simulink model "Scissor_Lift_4_Hydraulic_Actuator"  (Simulink 7.9)
settings: Solver=ode15s  StartTime=0.0  StopTime=10.0  MaxStep=1e-2  RelTol=1e-3  AbsTol=1e-4
PostLoadFcn:
  | warning off Simulink:Engine:OutputNotConnected
  | warning off mech2:compiler:topologyAnalysis:DanglingBlock
undefined symbols (not defined in the file): Local, Scissor_Lift_Param, X, Y, Z
libraries: sm_lib x48, Scissor_Parts_Lib x21, fl_lib x8, nesl_utility x7, sh_lib x4
(part 2 of 2)

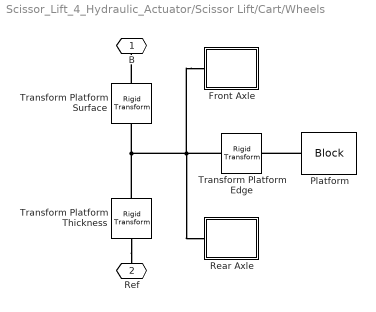
== system Scissor_Lift_4_Hydraulic_Actuator/Scissor Lift/Cart/Wheels ==
  Front Axle : Subsystem
  Platform : Scissor_Parts_Lib/Block  L=Scissor_Lift_Param.Cart.Platform.Width  W=Scissor_Lift_Param.Cart.Platform.Length  H=Scissor_Lift_Param.Cart.Platform.Height  z_ori=Local +Z  rho=Scissor_Lift_Param.Base_Block.Density  clr=Scissor_Lift_Param.Base_Block.Color  opc=Scissor_Lift_Param.Base_Block.Opacity
  Rear Axle : Subsystem
  Transform Platform Surface : sm_lib/Frames and  Transforms/Rigid  Transform  TranslationMethod=Cartesian  TranslationLengthUnit=cm  TranslationStandardAxis=+Y  TranslationStandardOffset=Scissor_Lift_Param.Cart.Platform.Height/2  TranslationCartesianOffset=[0 Scissor_Lift_Param.Cart.Platform.Height/2 0]  TranslationROffset=0  TranslationROffsetUnits=m  TranslationZOffset=0  TranslationZOffsetUnits=m  TranslationThetaOffset=0  TranslationThetaOffsetUnits=deg  RotationMethod=None  RotationAngleUnits=deg  RotationStandardAxis=+X  RotationAngle=90  RotationArbitraryAxis=[0 0 1]  FollAlignAxisA=+X  BaseAlignAxisA=+Y  FollAlignAxisB=+Y  BaseAlignAxisB=+Z  BlockFunction=simmechanics.library.frames_transforms.rigid_transform
  Transform Platform Thickness : sm_lib/Frames and  Transforms/Rigid  Transform  TranslationMethod=StandardAxis  TranslationLengthUnit=cm  TranslationStandardAxis=+Z  TranslationStandardOffset=Scissor_Lift_Param.Cart.Platform.Height/2  TranslationCartesianOffset=[0 0 0]  TranslationROffset=0  TranslationROffsetUnits=m  TranslationZOffset=0  TranslationZOffsetUnits=m  TranslationThetaOffset=0  TranslationThetaOffsetUnits=deg  RotationMethod=StandardAxis  RotationAngleUnits=deg  RotationStandardAxis=+X  RotationAngle=90  RotationArbitraryAxis=[0 0 1]  FollAlignAxisA=+X  BaseAlignAxisA=+Y  FollAlignAxisB=+Y  BaseAlignAxisB=+Z  BlockFunction=simmechanics.library.frames_transforms.rigid_transform
  Transform Platform Edge : sm_lib/Frames and  Transforms/Rigid  Transform  TranslationMethod=Cartesian  TranslationLengthUnit=cm  TranslationStandardAxis=+Z  TranslationStandardOffset=0  TranslationCartesianOffset=[Scissor_Lift_Param.Cart.Platform.Length 0 -Scissor_Lift_Param.Cart.Platform.Width]/2  TranslationROffset=0  TranslationROffsetUnits=m  TranslationZOffset=0  TranslationZOffsetUnits=m  TranslationThetaOffset=0  TranslationThetaOffsetUnits=deg  RotationMethod=None  RotationAngleUnits=deg  RotationStandardAxis=+X  RotationAngle=90  RotationArbitraryAxis=[0 0 1]  FollAlignAxisA=+X  BaseAlignAxisA=+Y  FollAlignAxisB=+Y  BaseAlignAxisB=+Z  BlockFunction=simmechanics.library.frames_transforms.rigid_transform
  " B" : PMIOPort  Port=1  Side=Right
  Ref : PMIOPort  Port=2  Side=Left
  connections:
  Transform Platform Surface/RConn1 -- " B"/RConn1
  Transform Platform Thickness/LConn1 -- Ref/RConn1
  Platform/LConn1 -- Transform Platform Edge/RConn1
  Front Axle/LConn1 -- Rear Axle/LConn1 -- Transform Platform Surface/LConn1 -- Transform Platform Thickness/RConn1 -- Transform Platform Edge/LConn1

== system Scissor_Lift_4_Hydraulic_Actuator/Scissor Lift/Actuator/Actuator/MS2G Intf ==
  Ideal Force Sensor : fl_lib/Mechanical/Mechanical Sensors/Ideal Force Sensor  v_Log=off  f_Log=off  LocalVarNames=|v|f  LocalVarDescs=|v|f  LocalVarLogging=[0 0]
  Ideal Translational Velocity Source : fl_lib/Mechanical/Mechanical Sources/Ideal Translational Velocity Source  v_Log=off  f_Log=off  LocalVarNames=|v|f  LocalVarDescs=|v|f  LocalVarLogging=[0 0]
  V : PMIOPort  Port=1  Side=Left
  F : PMIOPort  Port=2  Side=Right
  R : PMIOPort  Port=3  Side=Left
  C : PMIOPort  Port=4  Side=Right
  connections:
  V/RConn1 -- Ideal Translational Velocity Source/RConn1
  F/RConn1 -- Ideal Force Sensor/RConn2
  Ideal Force Sensor/LConn1 -- Ideal Translational Velocity Source/RConn2
  R/RConn1 -- Ideal Translational Velocity Source/LConn1
  Ideal Force Sensor/RConn1 -- C/RConn1

== system Scissor_Lift_4_Hydraulic_Actuator/Scissor Lift/Cart/Wheels/Front Axle ==
  Axle : Subsystem  mask(Axle){Ra=Scissor_Lift_Param.Cart.Axle.Radius, Wd=Scissor_Lift_Param.Cart.Axle.Wheel_Distance, Rr=Scissor_Lift_Param.Cart.Axle.Rim.Radius, Tr=Scissor_Lift_Param.Cart.Axle.Rim.Thickness, rho=Scissor_Lift_Param.Cart.Axle.Rim.Density, clr=Scissor_Lift_Param.Cart.Axle.Rim.Color}
      mask prompts: Ra "Axle radius (cm)"; Wd "Wheel distance (cm)"; Rr "Rim radius (cm)"; Tr "Rim thickness (cm)"; rho "Density (kg/m^3)"; clr "Color"
      mask TabNameString: Dimensions,Dimensions,Dimensions,Dimensions,Material Properties,Material Properties
      mask Display:
      | image(imread('sm_wlandgear_axle.png'));
      | port_label('LConn',1,'M');
      | port_label('RConn',1,'L');
      | port_label('RConn',2,'R');
  Axle-Tire A Revolute : sm_lib/Joints/Revolute Joint  SenseConstraintForceX=off  SenseConstraintForceY=off  SenseConstraintForceZ=off  SenseConstraintTorqueX=off  SenseConstraintTorqueY=off  SenseConstraintTorqueZ=off  ConstraintWrenchDir=FollowerOnBase  ConstraintWrenchFrame=BaseFrame  EquilibriumPosition=0  EquilibriumPositionUnits=rad  SpringStiffness=0  SpringStiffnessUnits=N*m/rad  DampingCoefficient=0  DampingCoefficientUnits=N*m/(rad/s)  ActuationMode=NoActuation  SensePosition=off  SenseVelocity=off  SenseAcceleration=off  SenseTorqueForce=off  PositionTargetValue=0  PositionTargetValueUnits=rad  PositionTargetSpecify=off  PositionTargetPriority=High  VelocityTargetValue=0  VelocityTargetValueUnits=rad/s  VelocityTargetSpecify=off  VelocityTargetPriority=High  BlockFunction=simmechanics.library.joints.revolute_joint
  Axle-Tire B Revolute : sm_lib/Joints/Revolute Joint  SenseConstraintForceX=off  SenseConstraintForceY=off  SenseConstraintForceZ=off  SenseConstraintTorqueX=off  SenseConstraintTorqueY=off  SenseConstraintTorqueZ=off  ConstraintWrenchDir=FollowerOnBase  ConstraintWrenchFrame=BaseFrame  EquilibriumPosition=0  EquilibriumPositionUnits=rad  SpringStiffness=0  SpringStiffnessUnits=N*m/rad  DampingCoefficient=0  DampingCoefficientUnits=N*m/(rad/s)  ActuationMode=NoActuation  SensePosition=off  SenseVelocity=off  SenseAcceleration=off  SenseTorqueForce=off  PositionTargetValue=0  PositionTargetValueUnits=rad  PositionTargetSpecify=off  PositionTargetPriority=High  VelocityTargetValue=0  VelocityTargetValueUnits=rad/s  VelocityTargetSpecify=off  VelocityTargetPriority=High  BlockFunction=simmechanics.library.joints.revolute_joint
  Tire A : Subsystem  mask(Tire){Rt=Scissor_Lift_Param.Cart.Axle.Tire.Radius, Rr=Scissor_Lift_Param.Cart.Axle.Rim.Radius, Tt=Scissor_Lift_Param.Cart.Axle.Tire.Thickness, rho=Scissor_Lift_Param.Cart.Axle.Tire.Density, clr=Scissor_Lift_Param.Cart.Axle.Tire.Color}
      mask prompts: Rt "Tire radius (cm)"; Rr "Rim radius (cm)"; Tt "Tire thickness (cm)"; rho "Density (kg/m^3)"; clr "Color"
      mask init:
      | theta = [(0:1:359) 0]'*pi/180;
      | unit_circle = [cos(theta), sin(theta)];
      | tire_sec = [Rt * unit_circle; Rr * flipud(unit_circle)];
      mask TabNameString: Dimensions,Dimensions,Dimensions,Material Properties,Material Properties
      mask Display:
      | image(imread('sm_wlandgear_tire.png'));
      | port_label('LConn',1,'C');
  Tire B : Subsystem  mask(Tire){Rt=Scissor_Lift_Param.Cart.Axle.Tire.Radius, Rr=Scissor_Lift_Param.Cart.Axle.Rim.Radius, Tt=Scissor_Lift_Param.Cart.Axle.Tire.Thickness, rho=Scissor_Lift_Param.Cart.Axle.Tire.Density, clr=Scissor_Lift_Param.Cart.Axle.Tire.Color}
      mask prompts: Rt "Tire radius (cm)"; Rr "Rim radius (cm)"; Tt "Tire thickness (cm)"; rho "Density (kg/m^3)"; clr "Color"
      mask init:
      | theta = [(0:1:359) 0]'*pi/180;
      | unit_circle = [cos(theta), sin(theta)];
      | tire_sec = [Rt * unit_circle; Rr * flipud(unit_circle)];
      mask TabNameString: Dimensions,Dimensions,Dimensions,Material Properties,Material Properties
      mask Display:
      | image(imread('sm_wlandgear_tire.png'));
      | port_label('LConn',1,'C');
  Transform Axle CG : sm_lib/Frames and  Transforms/Rigid  Transform  TranslationMethod=Cartesian  TranslationLengthUnit=cm  TranslationStandardAxis=+Z  TranslationStandardOffset=0  TranslationCartesianOffset=[Scissor_Lift_Param.Cart.Axle.Tire.Radius+Scissor_Lift_Param.Cart.Axle.Wheelbase -Scissor_Lift_Param.Cart.Axle.Tire.Radius 0]  TranslationROffset=0  TranslationROffsetUnits=m  TranslationZOffset=0  TranslationZOffsetUnits=m  TranslationThetaOffset=0  TranslationThetaOffsetUnits=deg  RotationMethod=None  RotationAngleUnits=deg  RotationStandardAxis=+X  RotationAngle=90  RotationArbitraryAxis=[0 0 1]  FollAlignAxisA=+X  BaseAlignAxisA=+Y  FollAlignAxisB=+Y  BaseAlignAxisB=+Z  BlockFunction=simmechanics.library.frames_transforms.rigid_transform
  P : PMIOPort  Port=1  Side=Left
  connections:
  Axle-Tire A Revolute/LConn1 -- Axle/RConn1
  Axle-Tire A Revolute/RConn1 -- Tire A/LConn1
  Axle-Tire B Revolute/LConn1 -- Axle/RConn2
  Axle-Tire B Revolute/RConn1 -- Tire B/LConn1
  Transform Axle CG/RConn1 -- Axle/LConn1
  P/RConn1 -- Transform Axle CG/LConn1

== system Scissor_Lift_4_Hydraulic_Actuator/Scissor Lift/Cart/Wheels/Rear Axle ==
  Axle : Subsystem  mask(Axle){Ra=Scissor_Lift_Param.Cart.Axle.Radius, Wd=Scissor_Lift_Param.Cart.Axle.Wheel_Distance, Rr=Scissor_Lift_Param.Cart.Axle.Rim.Radius, Tr=Scissor_Lift_Param.Cart.Axle.Rim.Thickness, rho=Scissor_Lift_Param.Cart.Axle.Rim.Density, clr=Scissor_Lift_Param.Cart.Axle.Rim.Color}
      mask prompts: Ra "Axle radius (cm)"; Wd "Wheel distance (cm)"; Rr "Rim radius (cm)"; Tr "Rim thickness (cm)"; rho "Density (kg/m^3)"; clr "Color"
      mask TabNameString: Dimensions,Dimensions,Dimensions,Dimensions,Material Properties,Material Properties
      mask Display:
      | image(imread('sm_wlandgear_axle.png'));
      | port_label('LConn',1,'M');
      | port_label('RConn',1,'L');
      | port_label('RConn',2,'R');
  Axle-Tire A Revolute : sm_lib/Joints/Revolute Joint  SenseConstraintForceX=off  SenseConstraintForceY=off  SenseConstraintForceZ=off  SenseConstraintTorqueX=off  SenseConstraintTorqueY=off  SenseConstraintTorqueZ=off  ConstraintWrenchDir=FollowerOnBase  ConstraintWrenchFrame=BaseFrame  EquilibriumPosition=0  EquilibriumPositionUnits=rad  SpringStiffness=0  SpringStiffnessUnits=N*m/rad  DampingCoefficient=0  DampingCoefficientUnits=N*m/(rad/s)  ActuationMode=NoActuation  SensePosition=off  SenseVelocity=off  SenseAcceleration=off  SenseTorqueForce=off  PositionTargetValue=0  PositionTargetValueUnits=rad  PositionTargetSpecify=off  PositionTargetPriority=High  VelocityTargetValue=0  VelocityTargetValueUnits=rad/s  VelocityTargetSpecify=off  VelocityTargetPriority=High  BlockFunction=simmechanics.library.joints.revolute_joint
  Axle-Tire B Revolute : sm_lib/Joints/Revolute Joint  SenseConstraintForceX=off  SenseConstraintForceY=off  SenseConstraintForceZ=off  SenseConstraintTorqueX=off  SenseConstraintTorqueY=off  SenseConstraintTorqueZ=off  ConstraintWrenchDir=FollowerOnBase  ConstraintWrenchFrame=BaseFrame  EquilibriumPosition=0  EquilibriumPositionUnits=rad  SpringStiffness=0  SpringStiffnessUnits=N*m/rad  DampingCoefficient=0  DampingCoefficientUnits=N*m/(rad/s)  ActuationMode=NoActuation  SensePosition=off  SenseVelocity=off  SenseAcceleration=off  SenseTorqueForce=off  PositionTargetValue=0  PositionTargetValueUnits=rad  PositionTargetSpecify=off  PositionTargetPriority=High  VelocityTargetValue=0  VelocityTargetValueUnits=rad/s  VelocityTargetSpecify=off  VelocityTargetPriority=High  BlockFunction=simmechanics.library.joints.revolute_joint
  Tire A : Subsystem  mask(Tire){Rt=Scissor_Lift_Param.Cart.Axle.Tire.Radius, Rr=Scissor_Lift_Param.Cart.Axle.Rim.Radius, Tt=Scissor_Lift_Param.Cart.Axle.Tire.Thickness, rho=Scissor_Lift_Param.Cart.Axle.Tire.Density, clr=Scissor_Lift_Param.Cart.Axle.Tire.Color}
      mask prompts: Rt "Tire radius (cm)"; Rr "Rim radius (cm)"; Tt "Tire thickness (cm)"; rho "Density (kg/m^3)"; clr "Color"
      mask init:
      | theta = [(0:1:359) 0]'*pi/180;
      | unit_circle = [cos(theta), sin(theta)];
      | tire_sec = [Rt * unit_circle; Rr * flipud(unit_circle)];
      mask TabNameString: Dimensions,Dimensions,Dimensions,Material Properties,Material Properties
      mask Display:
      | image(imread('sm_wlandgear_tire.png'));
      | port_label('LConn',1,'C');
  Tire B : Subsystem  mask(Tire){Rt=Scissor_Lift_Param.Cart.Axle.Tire.Radius, Rr=Scissor_Lift_Param.Cart.Axle.Rim.Radius, Tt=Scissor_Lift_Param.Cart.Axle.Tire.Thickness, rho=Scissor_Lift_Param.Cart.Axle.Tire.Density, clr=Scissor_Lift_Param.Cart.Axle.Tire.Color}
      mask prompts: Rt "Tire radius (cm)"; Rr "Rim radius (cm)"; Tt "Tire thickness (cm)"; rho "Density (kg/m^3)"; clr "Color"
      mask init:
      | theta = [(0:1:359) 0]'*pi/180;
      | unit_circle = [cos(theta), sin(theta)];
      | tire_sec = [Rt * unit_circle; Rr * flipud(unit_circle)];
      mask TabNameString: Dimensions,Dimensions,Dimensions,Material Properties,Material Properties
      mask Display:
      | image(imread('sm_wlandgear_tire.png'));
      | port_label('LConn',1,'C');
  Transform Axle CG : sm_lib/Frames and  Transforms/Rigid  Transform  TranslationMethod=Cartesian  TranslationLengthUnit=cm  TranslationStandardAxis=+Z  TranslationStandardOffset=0  TranslationCartesianOffset=[Scissor_Lift_Param.Cart.Axle.Tire.Radius -Scissor_Lift_Param.Cart.Axle.Tire.Radius 0]  TranslationROffset=0  TranslationROffsetUnits=m  TranslationZOffset=0  TranslationZOffsetUnits=m  TranslationThetaOffset=0  TranslationThetaOffsetUnits=deg  RotationMethod=None  RotationAngleUnits=deg  RotationStandardAxis=+X  RotationAngle=90  RotationArbitraryAxis=[0 0 1]  FollAlignAxisA=+X  BaseAlignAxisA=+Y  FollAlignAxisB=+Y  BaseAlignAxisB=+Z  BlockFunction=simmechanics.library.frames_transforms.rigid_transform
  P : PMIOPort  Port=1  Side=Left
  connections:
  P/RConn1 -- Transform Axle CG/LConn1
  Transform Axle CG/RConn1 -- Axle/LConn1
  Axle-Tire A Revolute/RConn1 -- Tire A/LConn1
  Axle-Tire B Revolute/RConn1 -- Tire B/LConn1
  Axle-Tire B Revolute/LConn1 -- Axle/RConn2
  Axle-Tire A Revolute/LConn1 -- Axle/RConn1

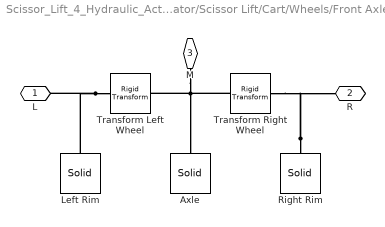
== system Scissor_Lift_4_Hydraulic_Actuator/Scissor Lift/Cart/Wheels/Front Axle/Axle ==
  Axle : sm_lib/Body Elements/Solid  InertiaType=CalculateFromGeometry  Mass=1  MassUnits=kg  CenterOfMass=[0 0 0]  CenterOfMassUnits=m  MomentsOfInertia=[1 1 1]  MomentsOfInertiaUnits=kg*m^2  ProductsOfInertia=[0 0 0]  ProductsOfInertiaUnits=kg*m^2  DensityBased=on  Density=rho  DensityUnits=kg/(m^3)  GraphicType=FromGeometry  MarkerShape=Sphere  MarkerSize=10  MarkerSizeUnits=m  GraphicVisPropType=SimpleVisualProperties  GraphicDiffuseColor=clr  GraphicSpecularColor=[0.5 0.5 0.5 1.0]  GraphicAmbientColor=[0.5 0.0 0.0 1.0]  GraphicEmissiveColor=[0.0 0.0 0.0 1.0]  GraphicShininess=75  GraphicOpacity=1.0  GeometryShape=Cylinder  RectangleSize=[1 1]  RectangleSizeUnits=m  BrickDimensions=[1 1 1]  BrickDimensionUnits=m  CylinderRadius=Ra  CylinderRadiusUnits=cm  CylinderLength=Wd  CylinderLengthUnits=cm  SphereRadius=1  SphereRadiusUnits=m  EllipsoidRadii=[1 1 1]  EllipsoidRadiiUnits=m  ExtrusionCrossSection=[1 1; -1 1; -1 -1; 1 -1]  ExtrusionCrossSectionUnits=m  ExtrusionLength=1  ExtrusionLengthUnits=m  PolygonNumSides=3  PolygonOuterRadius=1  PolygonOuterRadiusUnits=m  ExtGeomFileUnits=m  BlockFunction=simmechanics.library.body_elements.solid
  Left Rim : sm_lib/Body Elements/Solid  InertiaType=CalculateFromGeometry  Mass=1  MassUnits=kg  CenterOfMass=[0 0 0]  CenterOfMassUnits=m  MomentsOfInertia=[1 1 1]  MomentsOfInertiaUnits=kg*m^2  ProductsOfInertia=[0 0 0]  ProductsOfInertiaUnits=kg*m^2  DensityBased=on  Density=rho  DensityUnits=kg/(m^3)  GraphicType=FromGeometry  MarkerShape=Sphere  MarkerSize=10  MarkerSizeUnits=m  GraphicVisPropType=SimpleVisualProperties  GraphicDiffuseColor=clr  GraphicSpecularColor=[0.5 0.5 0.5 1.0]  GraphicAmbientColor=[0.5 0.0 0.0 1.0]  GraphicEmissiveColor=[0.0 0.0 0.0 1.0]  GraphicShininess=75  GraphicOpacity=1.0  GeometryShape=Cylinder  RectangleSize=[1 1]  RectangleSizeUnits=m  BrickDimensions=[1 1 1]  BrickDimensionUnits=m  CylinderRadius=Rr  CylinderRadiusUnits=cm  CylinderLength=Tr  CylinderLengthUnits=cm  SphereRadius=1  SphereRadiusUnits=m  EllipsoidRadii=[1 1 1]  EllipsoidRadiiUnits=m  ExtrusionCrossSection=[1 1; -1 1; -1 -1; 1 -1]  ExtrusionCrossSectionUnits=m  ExtrusionLength=1  ExtrusionLengthUnits=m  PolygonNumSides=3  PolygonOuterRadius=1  PolygonOuterRadiusUnits=m  ExtGeomFileUnits=m  BlockFunction=simmechanics.library.body_elements.solid
  "Right Rim " : sm_lib/Body Elements/Solid  InertiaType=CalculateFromGeometry  Mass=1  MassUnits=kg  CenterOfMass=[0 0 0]  CenterOfMassUnits=m  MomentsOfInertia=[1 1 1]  MomentsOfInertiaUnits=kg*m^2  ProductsOfInertia=[0 0 0]  ProductsOfInertiaUnits=kg*m^2  DensityBased=on  Density=rho  DensityUnits=kg/(m^3)  GraphicType=FromGeometry  MarkerShape=Sphere  MarkerSize=10  MarkerSizeUnits=m  GraphicVisPropType=SimpleVisualProperties  GraphicDiffuseColor=clr  GraphicSpecularColor=[0.5 0.5 0.5 1.0]  GraphicAmbientColor=[0.5 0.0 0.0 1.0]  GraphicEmissiveColor=[0.0 0.0 0.0 1.0]  GraphicShininess=75  GraphicOpacity=1.0  GeometryShape=Cylinder  RectangleSize=[1 1]  RectangleSizeUnits=m  BrickDimensions=[1 1 1]  BrickDimensionUnits=m  CylinderRadius=Rr  CylinderRadiusUnits=cm  CylinderLength=Tr  CylinderLengthUnits=cm  SphereRadius=1  SphereRadiusUnits=m  EllipsoidRadii=[1 1 1]  EllipsoidRadiiUnits=m  ExtrusionCrossSection=[1 1; -1 1; -1 -1; 1 -1]  ExtrusionCrossSectionUnits=m  ExtrusionLength=1  ExtrusionLengthUnits=m  PolygonNumSides=3  PolygonOuterRadius=1  PolygonOuterRadiusUnits=m  ExtGeomFileUnits=m  BlockFunction=simmechanics.library.body_elements.solid
  Transform Left Wheel : sm_lib/Frames and  Transforms/Rigid  Transform  TranslationMethod=StandardAxis  TranslationLengthUnit=cm  TranslationStandardAxis=-Z  TranslationStandardOffset=Wd/2 + Tr/2  TranslationCartesianOffset=[0 0 0]  TranslationROffset=0  TranslationROffsetUnits=m  TranslationZOffset=0  TranslationZOffsetUnits=m  TranslationThetaOffset=0  TranslationThetaOffsetUnits=deg  RotationMethod=None  RotationAngleUnits=deg  RotationStandardAxis=+Z  RotationAngle=0  RotationArbitraryAxis=[0 0 1]  FollAlignAxisA=+X  BaseAlignAxisA=+Y  FollAlignAxisB=+Y  BaseAlignAxisB=+Z  BlockFunction=simmechanics.library.frames_transforms.rigid_transform
  Transform Right Wheel : sm_lib/Frames and  Transforms/Rigid  Transform  TranslationMethod=StandardAxis  TranslationLengthUnit=cm  TranslationStandardAxis=+Z  TranslationStandardOffset=Wd/2 + Tr/2  TranslationCartesianOffset=[0 0 0]  TranslationROffset=0  TranslationROffsetUnits=m  TranslationZOffset=0  TranslationZOffsetUnits=m  TranslationThetaOffset=0  TranslationThetaOffsetUnits=deg  RotationMethod=None  RotationAngleUnits=deg  RotationStandardAxis=+Z  RotationAngle=0  RotationArbitraryAxis=[0 0 1]  FollAlignAxisA=+X  BaseAlignAxisA=+Y  FollAlignAxisB=+Y  BaseAlignAxisB=+Z  BlockFunction=simmechanics.library.frames_transforms.rigid_transform
  L : PMIOPort  Port=1  Side=Right
  R : PMIOPort  Port=2  Side=Right
  M : PMIOPort  Port=3  Side=Left
  connections:
  "Right Rim "/RConn1 -- Transform Right Wheel/RConn1 -- R/RConn1
  M/RConn1 -- Axle/RConn1 -- Transform Right Wheel/LConn1 -- Transform Left Wheel/LConn1
  Transform Left Wheel/RConn1 -- Left Rim/RConn1 -- L/RConn1

== system Scissor_Lift_4_Hydraulic_Actuator/Scissor Lift/Cart/Wheels/Front Axle/Tire A ==
  Tire : sm_lib/Body Elements/Solid  InertiaType=CalculateFromGeometry  Mass=1  MassUnits=kg  CenterOfMass=[0 0 0]  CenterOfMassUnits=m  MomentsOfInertia=[1 1 1]  MomentsOfInertiaUnits=kg*m^2  ProductsOfInertia=[0 0 0]  ProductsOfInertiaUnits=kg*m^2  DensityBased=on  Density=rho  DensityUnits=kg/(m^3)  GraphicType=FromGeometry  MarkerShape=Sphere  MarkerSize=10  MarkerSizeUnits=m  GraphicVisPropType=SimpleVisualProperties  GraphicDiffuseColor=clr  GraphicSpecularColor=[0.5 0.5 0.5 1.0]  GraphicAmbientColor=[0.5 0.0 0.0 1.0]  GraphicEmissiveColor=[0.0 0.0 0.0 1.0]  GraphicShininess=75  GraphicOpacity=1.0  GeometryShape=GeneralExtrusion  RectangleSize=[1 1]  RectangleSizeUnits=m  BrickDimensions=[1 1 1]  BrickDimensionUnits=m  CylinderRadius=1  CylinderRadiusUnits=m  CylinderLength=1  CylinderLengthUnits=m  SphereRadius=1  SphereRadiusUnits=m  EllipsoidRadii=[1 1 1]  EllipsoidRadiiUnits=m  ExtrusionCrossSection=tire_sec  ExtrusionCrossSectionUnits=cm  ExtrusionLength=Tt  ExtrusionLengthUnits=cm  PolygonNumSides=3  PolygonOuterRadius=1  PolygonOuterRadiusUnits=m  ExtGeomFileUnits=m  BlockFunction=simmechanics.library.body_elements.solid
  C : PMIOPort  Port=1  Side=Left
  connections:
  Tire/RConn1 -- C/RConn1

== system Scissor_Lift_4_Hydraulic_Actuator/Scissor Lift/Cart/Wheels/Front Axle/Tire B ==
  Tire : sm_lib/Body Elements/Solid  InertiaType=CalculateFromGeometry  Mass=1  MassUnits=kg  CenterOfMass=[0 0 0]  CenterOfMassUnits=m  MomentsOfInertia=[1 1 1]  MomentsOfInertiaUnits=kg*m^2  ProductsOfInertia=[0 0 0]  ProductsOfInertiaUnits=kg*m^2  DensityBased=on  Density=rho  DensityUnits=kg/(m^3)  GraphicType=FromGeometry  MarkerShape=Sphere  MarkerSize=10  MarkerSizeUnits=m  GraphicVisPropType=SimpleVisualProperties  GraphicDiffuseColor=clr  GraphicSpecularColor=[0.5 0.5 0.5 1.0]  GraphicAmbientColor=[0.5 0.0 0.0 1.0]  GraphicEmissiveColor=[0.0 0.0 0.0 1.0]  GraphicShininess=75  GraphicOpacity=1.0  GeometryShape=GeneralExtrusion  RectangleSize=[1 1]  RectangleSizeUnits=m  BrickDimensions=[1 1 1]  BrickDimensionUnits=m  CylinderRadius=1  CylinderRadiusUnits=m  CylinderLength=1  CylinderLengthUnits=m  SphereRadius=1  SphereRadiusUnits=m  EllipsoidRadii=[1 1 1]  EllipsoidRadiiUnits=m  ExtrusionCrossSection=tire_sec  ExtrusionCrossSectionUnits=cm  ExtrusionLength=Tt  ExtrusionLengthUnits=cm  PolygonNumSides=3  PolygonOuterRadius=1  PolygonOuterRadiusUnits=m  ExtGeomFileUnits=m  BlockFunction=simmechanics.library.body_elements.solid
  C : PMIOPort  Port=1  Side=Left
  connections:
  Tire/RConn1 -- C/RConn1

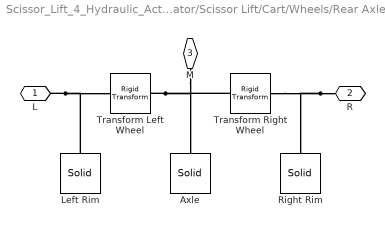
== system Scissor_Lift_4_Hydraulic_Actuator/Scissor Lift/Cart/Wheels/Rear Axle/Axle ==
  Axle : sm_lib/Body Elements/Solid  InertiaType=CalculateFromGeometry  Mass=1  MassUnits=kg  CenterOfMass=[0 0 0]  CenterOfMassUnits=m  MomentsOfInertia=[1 1 1]  MomentsOfInertiaUnits=kg*m^2  ProductsOfInertia=[0 0 0]  ProductsOfInertiaUnits=kg*m^2  DensityBased=on  Density=rho  DensityUnits=kg/(m^3)  GraphicType=FromGeometry  MarkerShape=Sphere  MarkerSize=10  MarkerSizeUnits=m  GraphicVisPropType=SimpleVisualProperties  GraphicDiffuseColor=clr  GraphicSpecularColor=[0.5 0.5 0.5 1.0]  GraphicAmbientColor=[0.5 0.0 0.0 1.0]  GraphicEmissiveColor=[0.0 0.0 0.0 1.0]  GraphicShininess=75  GraphicOpacity=1.0  GeometryShape=Cylinder  RectangleSize=[1 1]  RectangleSizeUnits=m  BrickDimensions=[1 1 1]  BrickDimensionUnits=m  CylinderRadius=Ra  CylinderRadiusUnits=cm  CylinderLength=Wd  CylinderLengthUnits=cm  SphereRadius=1  SphereRadiusUnits=m  EllipsoidRadii=[1 1 1]  EllipsoidRadiiUnits=m  ExtrusionCrossSection=[1 1; -1 1; -1 -1; 1 -1]  ExtrusionCrossSectionUnits=m  ExtrusionLength=1  ExtrusionLengthUnits=m  PolygonNumSides=3  PolygonOuterRadius=1  PolygonOuterRadiusUnits=m  ExtGeomFileUnits=m  BlockFunction=simmechanics.library.body_elements.solid
  Left Rim : sm_lib/Body Elements/Solid  InertiaType=CalculateFromGeometry  Mass=1  MassUnits=kg  CenterOfMass=[0 0 0]  CenterOfMassUnits=m  MomentsOfInertia=[1 1 1]  MomentsOfInertiaUnits=kg*m^2  ProductsOfInertia=[0 0 0]  ProductsOfInertiaUnits=kg*m^2  DensityBased=on  Density=rho  DensityUnits=kg/(m^3)  GraphicType=FromGeometry  MarkerShape=Sphere  MarkerSize=10  MarkerSizeUnits=m  GraphicVisPropType=SimpleVisualProperties  GraphicDiffuseColor=clr  GraphicSpecularColor=[0.5 0.5 0.5 1.0]  GraphicAmbientColor=[0.5 0.0 0.0 1.0]  GraphicEmissiveColor=[0.0 0.0 0.0 1.0]  GraphicShininess=75  GraphicOpacity=1.0  GeometryShape=Cylinder  RectangleSize=[1 1]  RectangleSizeUnits=m  BrickDimensions=[1 1 1]  BrickDimensionUnits=m  CylinderRadius=Rr  CylinderRadiusUnits=cm  CylinderLength=Tr  CylinderLengthUnits=cm  SphereRadius=1  SphereRadiusUnits=m  EllipsoidRadii=[1 1 1]  EllipsoidRadiiUnits=m  ExtrusionCrossSection=[1 1; -1 1; -1 -1; 1 -1]  ExtrusionCrossSectionUnits=m  ExtrusionLength=1  ExtrusionLengthUnits=m  PolygonNumSides=3  PolygonOuterRadius=1  PolygonOuterRadiusUnits=m  ExtGeomFileUnits=m  BlockFunction=simmechanics.library.body_elements.solid
  "Right Rim " : sm_lib/Body Elements/Solid  InertiaType=CalculateFromGeometry  Mass=1  MassUnits=kg  CenterOfMass=[0 0 0]  CenterOfMassUnits=m  MomentsOfInertia=[1 1 1]  MomentsOfInertiaUnits=kg*m^2  ProductsOfInertia=[0 0 0]  ProductsOfInertiaUnits=kg*m^2  DensityBased=on  Density=rho  DensityUnits=kg/(m^3)  GraphicType=FromGeometry  MarkerShape=Sphere  MarkerSize=10  MarkerSizeUnits=m  GraphicVisPropType=SimpleVisualProperties  GraphicDiffuseColor=clr  GraphicSpecularColor=[0.5 0.5 0.5 1.0]  GraphicAmbientColor=[0.5 0.0 0.0 1.0]  GraphicEmissiveColor=[0.0 0.0 0.0 1.0]  GraphicShininess=75  GraphicOpacity=1.0  GeometryShape=Cylinder  RectangleSize=[1 1]  RectangleSizeUnits=m  BrickDimensions=[1 1 1]  BrickDimensionUnits=m  CylinderRadius=Rr  CylinderRadiusUnits=cm  CylinderLength=Tr  CylinderLengthUnits=cm  SphereRadius=1  SphereRadiusUnits=m  EllipsoidRadii=[1 1 1]  EllipsoidRadiiUnits=m  ExtrusionCrossSection=[1 1; -1 1; -1 -1; 1 -1]  ExtrusionCrossSectionUnits=m  ExtrusionLength=1  ExtrusionLengthUnits=m  PolygonNumSides=3  PolygonOuterRadius=1  PolygonOuterRadiusUnits=m  ExtGeomFileUnits=m  BlockFunction=simmechanics.library.body_elements.solid
  Transform Left Wheel : sm_lib/Frames and  Transforms/Rigid  Transform  TranslationMethod=StandardAxis  TranslationLengthUnit=cm  TranslationStandardAxis=-Z  TranslationStandardOffset=Wd/2 + Tr/2  TranslationCartesianOffset=[0 0 0]  TranslationROffset=0  TranslationROffsetUnits=m  TranslationZOffset=0  TranslationZOffsetUnits=m  TranslationThetaOffset=0  TranslationThetaOffsetUnits=deg  RotationMethod=None  RotationAngleUnits=deg  RotationStandardAxis=+Z  RotationAngle=0  RotationArbitraryAxis=[0 0 1]  FollAlignAxisA=+X  BaseAlignAxisA=+Y  FollAlignAxisB=+Y  BaseAlignAxisB=+Z  BlockFunction=simmechanics.library.frames_transforms.rigid_transform
  Transform Right Wheel : sm_lib/Frames and  Transforms/Rigid  Transform  TranslationMethod=StandardAxis  TranslationLengthUnit=cm  TranslationStandardAxis=+Z  TranslationStandardOffset=Wd/2 + Tr/2  TranslationCartesianOffset=[0 0 0]  TranslationROffset=0  TranslationROffsetUnits=m  TranslationZOffset=0  TranslationZOffsetUnits=m  TranslationThetaOffset=0  TranslationThetaOffsetUnits=deg  RotationMethod=None  RotationAngleUnits=deg  RotationStandardAxis=+Z  RotationAngle=0  RotationArbitraryAxis=[0 0 1]  FollAlignAxisA=+X  BaseAlignAxisA=+Y  FollAlignAxisB=+Y  BaseAlignAxisB=+Z  BlockFunction=simmechanics.library.frames_transforms.rigid_transform
  L : PMIOPort  Port=1  Side=Right
  R : PMIOPort  Port=2  Side=Right
  M : PMIOPort  Port=3  Side=Left
  connections:
  L/RConn1 -- Left Rim/RConn1 -- Transform Left Wheel/RConn1
  Transform Left Wheel/LConn1 -- Transform Right Wheel/LConn1 -- Axle/RConn1 -- M/RConn1
  R/RConn1 -- Transform Right Wheel/RConn1 -- "Right Rim "/RConn1

== system Scissor_Lift_4_Hydraulic_Actuator/Scissor Lift/Cart/Wheels/Rear Axle/Tire A ==
  Tire : sm_lib/Body Elements/Solid  InertiaType=CalculateFromGeometry  Mass=1  MassUnits=kg  CenterOfMass=[0 0 0]  CenterOfMassUnits=m  MomentsOfInertia=[1 1 1]  MomentsOfInertiaUnits=kg*m^2  ProductsOfInertia=[0 0 0]  ProductsOfInertiaUnits=kg*m^2  DensityBased=on  Density=rho  DensityUnits=kg/(m^3)  GraphicType=FromGeometry  MarkerShape=Sphere  MarkerSize=10  MarkerSizeUnits=m  GraphicVisPropType=SimpleVisualProperties  GraphicDiffuseColor=clr  GraphicSpecularColor=[0.5 0.5 0.5 1.0]  GraphicAmbientColor=[0.5 0.0 0.0 1.0]  GraphicEmissiveColor=[0.0 0.0 0.0 1.0]  GraphicShininess=75  GraphicOpacity=1.0  GeometryShape=GeneralExtrusion  RectangleSize=[1 1]  RectangleSizeUnits=m  BrickDimensions=[1 1 1]  BrickDimensionUnits=m  CylinderRadius=1  CylinderRadiusUnits=m  CylinderLength=1  CylinderLengthUnits=m  SphereRadius=1  SphereRadiusUnits=m  EllipsoidRadii=[1 1 1]  EllipsoidRadiiUnits=m  ExtrusionCrossSection=tire_sec  ExtrusionCrossSectionUnits=cm  ExtrusionLength=Tt  ExtrusionLengthUnits=cm  PolygonNumSides=3  PolygonOuterRadius=1  PolygonOuterRadiusUnits=m  ExtGeomFileUnits=m  BlockFunction=simmechanics.library.body_elements.solid
  C : PMIOPort  Port=1  Side=Left
  connections:
  Tire/RConn1 -- C/RConn1

== system Scissor_Lift_4_Hydraulic_Actuator/Scissor Lift/Cart/Wheels/Rear Axle/Tire B ==
  Tire : sm_lib/Body Elements/Solid  InertiaType=CalculateFromGeometry  Mass=1  MassUnits=kg  CenterOfMass=[0 0 0]  CenterOfMassUnits=m  MomentsOfInertia=[1 1 1]  MomentsOfInertiaUnits=kg*m^2  ProductsOfInertia=[0 0 0]  ProductsOfInertiaUnits=kg*m^2  DensityBased=on  Density=rho  DensityUnits=kg/(m^3)  GraphicType=FromGeometry  MarkerShape=Sphere  MarkerSize=10  MarkerSizeUnits=m  GraphicVisPropType=SimpleVisualProperties  GraphicDiffuseColor=clr  GraphicSpecularColor=[0.5 0.5 0.5 1.0]  GraphicAmbientColor=[0.5 0.0 0.0 1.0]  GraphicEmissiveColor=[0.0 0.0 0.0 1.0]  GraphicShininess=75  GraphicOpacity=1.0  GeometryShape=GeneralExtrusion  RectangleSize=[1 1]  RectangleSizeUnits=m  BrickDimensions=[1 1 1]  BrickDimensionUnits=m  CylinderRadius=1  CylinderRadiusUnits=m  CylinderLength=1  CylinderLengthUnits=m  SphereRadius=1  SphereRadiusUnits=m  EllipsoidRadii=[1 1 1]  EllipsoidRadiiUnits=m  ExtrusionCrossSection=tire_sec  ExtrusionCrossSectionUnits=cm  ExtrusionLength=Tt  ExtrusionLengthUnits=cm  PolygonNumSides=3  PolygonOuterRadius=1  PolygonOuterRadiusUnits=m  ExtGeomFileUnits=m  BlockFunction=simmechanics.library.body_elements.solid
  C : PMIOPort  Port=1  Side=Left
  connections:
  Tire/RConn1 -- C/RConn1
